simulink model "sistemaControlloPID"  (R2021a)
settings: Solver=VariableStepAuto  StartTime=0.0  StopTime=10  RelTol=1e-3
values from neighbouring files (symbols this model uses):
  b = 0.1    [controlloPID.m]    (also in modello_CA.m)
  g = 9.8    [controlloPID.m]    (also in modello2.m = 9.81; modello_CA.m = 9.81)
  i = 0.006    [controlloPID.m]    (also in modello_CA.m = 0.00030246)
  l = 0.3    [controlloPID.m]    (also in modello2.m = 0.071; modello_CA.m = 0.071)
  M = 0.5    [controlloPID.m]    (also in modello2.m = 0.04; modello_CA.m = 0.04)
  m = 0.2    [controlloPID.m]    (also in modello2.m = 0.06; modello_CA.m = 0.06)
  p0 = 0    [controlloPID.m]    (also in modello_CA.m)
  theta0 = 1.5    [controlloPID.m]    (also in modello_CA.m = rand())
  velocita0 = 0    [controlloPID.m]    (also in modello_CA.m)
  w0 = 2    [controlloPID.m]    (also in modello_CA.m = rand())
libraries: pid_lib x1
settings Model: Creator=adolfocafaro  LastModifiedBy=adolfocafaro

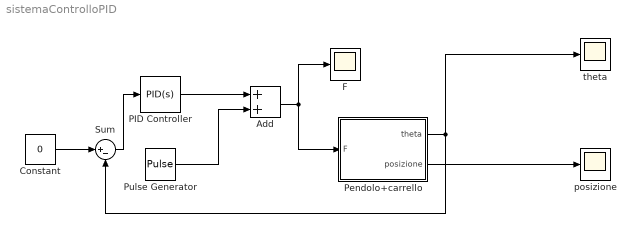
== system sistemaControlloPID ==
  Add : Sum
  Constant : Constant  Value=0
  F : Scope
  PID Controller : pid_lib/PID Controller  Controller=PID  Form=Parallel  TimeDomain=Continuous-time  UseExternalTs=off  SampleTime=-1  IntegratorMethod=Forward Euler  FilterMethod=Forward Euler  ControllerParametersSource=internal  P=100  I=1  D=20  UseFilter=on  N=100  TunerSelectOption=Transfer Function Based (PID Tuner App)  InitialConditionSource=internal  InitialConditionForIntegrator=0  InitialConditionForFilter=0  DifferentiatorICPrevScaledInput=0  ExternalReset=none  TrackingMode=off  Kt=1  LimitOutput=off  SatLimitsSource=internal  UpperSaturationLimit=inf  LowerSaturationLimit=-inf  LinearizeAsGain=on  AntiWindupMode=none  Kb=1  POutMin=[]  POutMax=[]  IOutMin=[]  IOutMax=[]  DOutMin=[]  DOutMax=[]  NOutMin=[]  NOutMax=[]  SumOutMin=[]  SumOutMax=[]  SaturationOutMin=[]  SaturationOutMax=[]  PParamMin=[]  PParamMax=[]  IParamMin=[]  IParamMax=[]  DParamMin=[]  DParamMax=[]  NParamMin=[]  NParamMax=[]  KbParamMin=[]  KbParamMax=[]  KtParamMin=[]  KtParamMax=[]  KbOutMin=[]  KbOutMax=[]  KtOutMin=[]  KtOutMax=[]  IntegratorOutMin=[]  IntegratorOutMax=[]  FilterOutMin=[]  FilterOutMax=[]  SumI1OutMin=[]  SumI1OutMax=[]  SumI2OutMin=[]  SumI2OutMax=[]  SumI3OutMin=[]  SumI3OutMax=[]  SumI4OutMin=[]  SumI4OutMax=[]  SumDOutMin=[]  SumDOutMax=[]  DifferentiatorOutMin=[]  DifferentiatorOutMax=[]  FilterDiffOutCoefMin=[]  FilterDiffOutCoefMax=[]  ReciprocalOutMin=[]  ReciprocalOutMax=[]  SumDenOutMin=[]  SumDenOutMax=[]  SumNumOutMin=[]  SumNumOutMax=[]  DivideOutMin=[]  DivideOutMax=[]  UdiffTsProdOutMin=[]  UdiffTsProdOutMax=[]  NTsProdOutMin=[]  NTsProdOutMax=[]  UintegralTsProdOutMin=[]  UintegralTsProdOutMax=[]  UngainTsProdOutMin=[]  UngainTsProdOutMax=[]  IntegratorContinuousStateAttributes=''  IntegratorStateMustResolveToSignalObject=off  IntegratorRTWStateStorageClass=Auto  FilterContinuousStateAttributes=''  FilterStateMustResolveToSignalObject=off  FilterRTWStateStorageClass=Auto  ParallelPVariant=InternalParameters  IdealPVariant=Disabled  IVariant=InternalParameters  DVariant=InternalParameters  IntegratorVariant=Continuous  SatVariant=Disabled  AWVariant=Passthrough  PCopyVariant=Disabled  TRVariant=Disabled  FdbkBlocksVariant=Forward  IdealPFdbkVariant=Disabled  SatFdbkVariant=Disabled  DerivativeFilterVariant=ContFilter  NVariant=InternalParameters  NCopyVariant=Disabled  FilterICVariant=InternalICsFilter  IntegratorICVariant=InternalICs  ExternalResetVariant=Disabled  TRSumVariant=Passthrough  SumFdbkVariant=Disabled  SumVariant=Sum_PID  TsampFilterVariant=InternalTs  TsampNgainVariant=Passthrough  TsampIntegralVariant=Passthrough  ExternalSaturationOutDataTypeStr=Inherit: Same as second input
  "Pendolo+carrello " : Subsystem
  Pulse Generator : DiscretePulseGenerator  PulseType=Time based  Period=10  PulseWidth=5
  Sum : Sum  Inputs=|+-
  posizione : Scope
  theta : Scope
  wires:
  "Pendolo+carrello "/1(theta) -> theta/1, Sum/2
  "Pendolo+carrello "/2(posizione) -> posizione/1
  Sum/1 -> PID Controller/1
  Constant/1 -> Sum/1
  PID Controller/1 -> Add/1
  Pulse Generator/1 -> Add/2
  Add/1 -> "Pendolo+carrello "/1(F), F/1

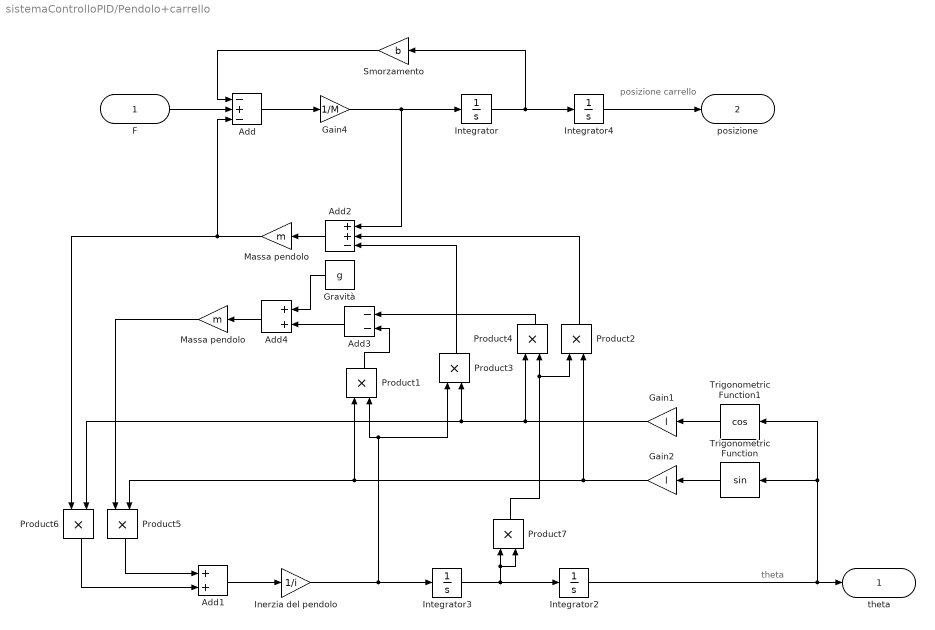
== system sistemaControlloPID/Pendolo+carrello  ==
  note: theta
  note: posizione carrello
  F : Inport
  Add : Sum  Inputs=-+-
  Add1 : Sum
  Add2 : Sum  Inputs=++-
  Add3 : Sum  Inputs=--
  Add4 : Sum
  Gain1 : Gain  Gain=l
  Gain2 : Gain  Gain=l
  Gain4 : Gain  Gain=1/M
  Gravità : Constant  Value=g
  Inerzia del pendolo : Gain  Gain=1/i
  Integrator : Integrator  InitialCondition=velocita0
  Integrator2 : Integrator  InitialCondition=theta0
  Integrator3 : Integrator  InitialCondition=w0
  Integrator4 : Integrator  InitialCondition=p0
  Massa pendolo : Gain  Gain=m
  "Massa pendolo " : Gain  Gain=m
  Product{1..7} (7 alike) : Product
  Smorzamento : Gain  Gain=b
  Trigonometric Function : Trigonometry
  Trigonometric Function1 : Trigonometry  Operator=cos
  theta : Outport
  posizione : Outport  Port=2
  wires:
  Trigonometric Function1/1 -> Gain1/1
  Product2/1 -> Add2/2
  Product7/1 -> Product2/1, Product4/2
  Integrator4/1 -> posizione/1
  Product6/1 -> Add1/2
  Product5/1 -> Add1/1
  Integrator3/1 -> Product7/2, Product7/1, Integrator2/1
  Product3/1 -> Add2/3
  Gravità/1 -> Add4/1
  Gain2/1 -> Product2/2, Product5/2, Product1/1
  Add/1 -> Gain4/1
  Trigonometric Function/1 -> Gain2/1
  Integrator2/1 -> theta/1, Trigonometric Function1/1, Trigonometric Function/1
  Add4/1 -> "Massa pendolo "/1
  Product4/1 -> Add3/1
  Add1/1 -> Inerzia del pendolo/1
  Inerzia del pendolo/1 -> Integrator3/1, Product3/1, Product1/2
  Massa pendolo/1 -> Add/3, Product6/1
  Smorzamento/1 -> Add/1
  Add2/1 -> Massa pendolo/1
  Product1/1 -> Add3/2
  F/1 -> Add/2
  Integrator/1 -> Smorzamento/1, Integrator4/1
  Add3/1 -> Add4/2
  "Massa pendolo "/1 -> Product5/1
  Gain1/1 -> Product3/2, Product6/2, Product4/1
  Gain4/1 -> Add2/1, Integrator/1
